simulink subsystem "SystemInputsSimFOCSL"  (R2024b)
settings: Solver=VariableStepAuto  StartTime=0.0  StopTime=10.0  RelTol=1e-3
undefined symbols (not defined in the file or in its folder): pmsm
libraries: simulink x1
settings Model: Creator=The MathWorks, Inc.  LastModifiedBy=snarayan
settings RTWCC: GPUComputeCapability=3.5  LargeConstantGeneration=WriteOnlyDNNConstantsToDataFiles

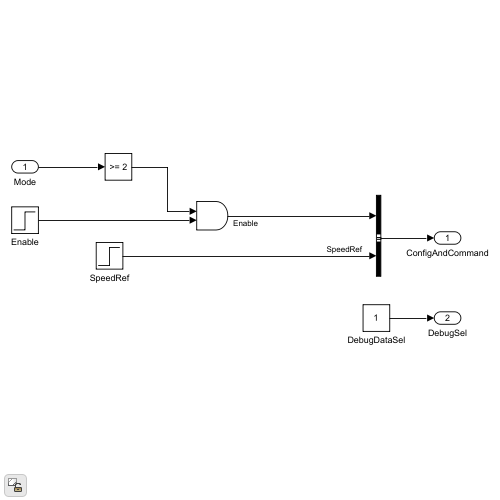
[thumbnail: Simulink's stored preview of the top-level diagram]
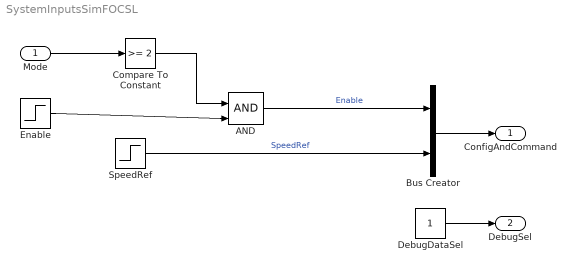
== system SystemInputsSimFOCSL ==
  Mode : Inport
  AND : Logic  IconShape=distinctive  AllPortsSameDT=off  OutDataTypeStr=boolean
  Bus Creator : BusCreator  Inputs=2
  Compare To Constant : simulink/Logic and Bit Operations/Compare To Constant  relop=>=  const=2  OutDataTypeStr=boolean
  DebugDataSel : Constant  OutDataTypeStr=uint8
  Enable : Step  Time=0.5  OutDataTypeStr=single
  SpeedRef : Step  Time=13  Before=pmsm.N_rated * 0.21  After=pmsm.N_rated * 0.8  OutDataTypeStr=single
  ConfigAndCommand : Outport
  DebugSel : Outport  Port=2
  wires:
  DebugDataSel/1 -> DebugSel/1
  SpeedRef/1 -> Bus Creator/2  "SpeedRef"
  Bus Creator/1 -> ConfigAndCommand/1
  AND/1 -> Bus Creator/1  "Enable"
  Mode/1 -> Compare To Constant/1
  Enable/1 -> AND/2
  Compare To Constant/1 -> AND/1
